simulink model "sixDOF"  (R2023b)
settings: Solver=FixedStepAuto  StartTime=0.0  StopTime=500  FixedStep=time_step  RelTol=1e-3
model workspace: external: MAT-File params.mat (data not in the file)
values from neighbouring files (symbols this model uses):
  currentmass = 0.3    [params.mat]
  drymass = 0.25    [params.mat]    (also in setRocketConstants.m)
  earth_mass = 5.9722e+24    [params.mat]
  earth_radius = 6371852    [params.mat]
  G = 6.6743e-11    [params.mat]
  motor = [0 0.002 0.05 0.1 0.2 0.274 0.292 0.31 0.32 0.33 0.34 0.35 ... (64 elements, 32x2)]    [params.mat]    (also in setRocketConstants.m = table2array(readtable('motor.txt')))
  q0 = [1 0 0 0]    [params.mat]    (also in setRocketConstants.m = [1; 0; 0; 0])
  qBody2IMU = [1 0 0 0]    [params.mat]
  time_step = 0.01    [params.mat]
  wetmass = 0.3    [params.mat]    (also in setRocketConstants.m)
  x0 = [0 0 0 0 0 0 0 0 0]    [params.mat]    (also in setRocketConstants.m = [0; 0; 0; 0; 0; 0; 0; 0; 0])
libraries: aerolibutil x6, shared6dof x1, aerolibnav x1
settings Model: Creator=roger  LastModifiedBy=roger

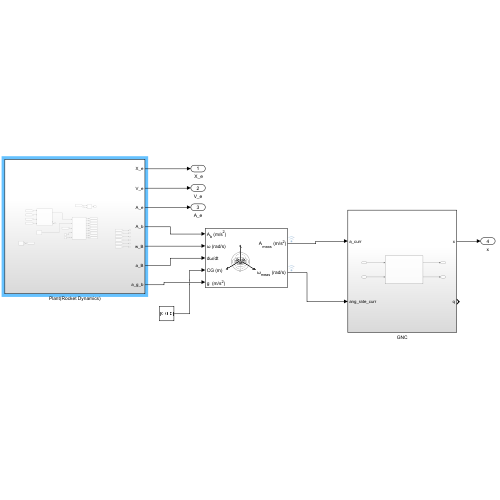
[thumbnail: Simulink's stored preview of the top-level diagram]
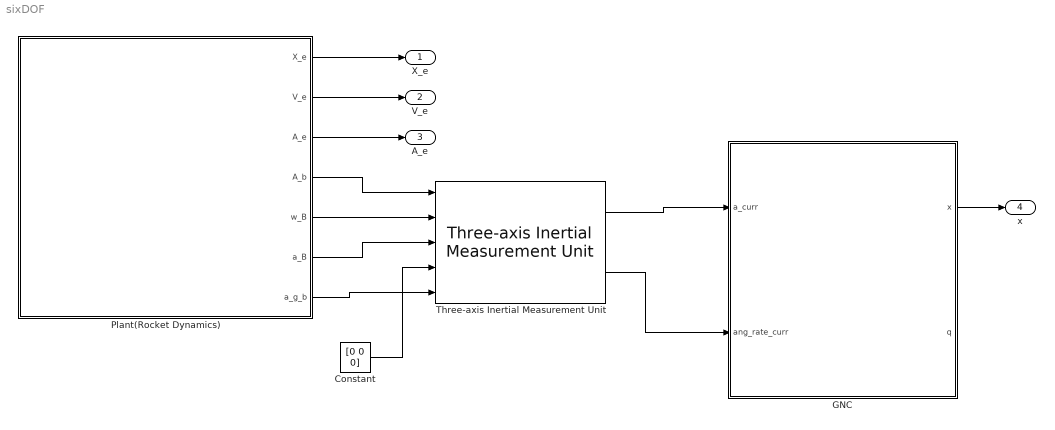
== system sixDOF ==
  Constant : Constant  Value=[0 0 0]
  GNC : Subsystem
  Plant(Rocket Dynamics) : Subsystem
  Three-axis Inertial Measurement Unit : aerolibnav/Three-axis Inertial Measurement Unit  units=Metric (MKS)  imu=[0 0 0]  i_Ts=0.01  dtype_a=on  w_a=190  z_a=0.707  a_sf_cc=[1 0 0; 0 1 0; 0 0 1]  a_bias=[0 0 0]  a_sat="[-inf  -inf  -inf  inf inf inf]"  dtype_g=on  w_g=190  z_g=0.707  g_sf_cc=[1 0 0; 0 1 0; 0 0 1]  g_bias=[0 0 0]  g_sens=[0 0 0]  g_sat="[-inf  -inf  -inf  inf inf inf]"  i_rand=off  i_seeds=[23093 23094 23095 23096 23097 23098]  i_pow=[0.001 0.001 0.001 0.0001 0.0001 0.0001]
  " X_e" : Outport
  V_e : Outport  Port=2
  A_e : Outport  Port=3
  x : Outport  Port=4
  wires:
  Constant/1 -> Three-axis Inertial Measurement Unit/4
  Plant(Rocket Dynamics)/3(A_e) -> A_e/1
  Plant(Rocket Dynamics)/5(w_B) -> Three-axis Inertial Measurement Unit/2
  Plant(Rocket Dynamics)/6(a_B) -> Three-axis Inertial Measurement Unit/3
  Plant(Rocket Dynamics)/4(A_b) -> Three-axis Inertial Measurement Unit/1
  Plant(Rocket Dynamics)/7(a_g_b) -> Three-axis Inertial Measurement Unit/5
  Plant(Rocket Dynamics)/1(X_e) -> " X_e"/1
  Plant(Rocket Dynamics)/2(V_e) -> V_e/1
  Three-axis Inertial Measurement Unit/1 -> GNC/1(a_curr)
  Three-axis Inertial Measurement Unit/2 -> GNC/2(ang_rate_curr)
  GNC/1(x) -> x/1

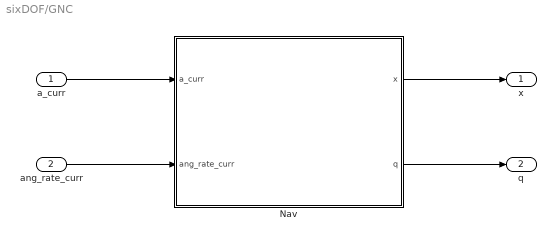
== system sixDOF/GNC ==
  a_curr : Inport
  ang_rate_curr : Inport  Port=2
  Nav : Subsystem
  x : Outport
  q : Outport  Port=2
  wires:
  a_curr/1 -> Nav/1(a_curr)
  ang_rate_curr/1 -> Nav/2(ang_rate_curr)
  Nav/1(x) -> x/1
  Nav/2(q) -> q/1

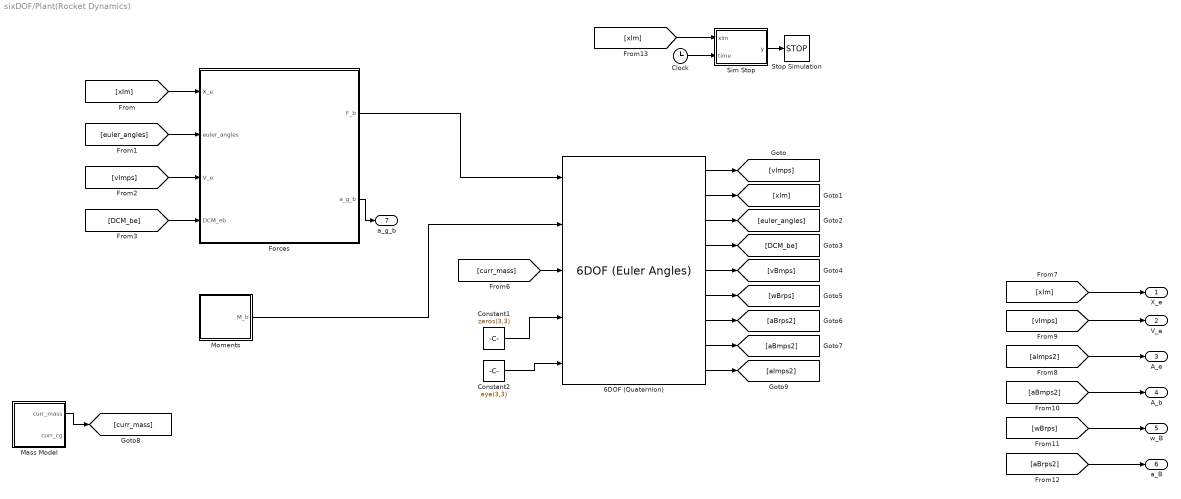
== system sixDOF/Plant(Rocket Dynamics) ==
  "6DOF (Quaternion) " : shared6dof/6DOF (Euler Angles)  units=Metric (MKS)  mtype=Custom Variable  rep=Quaternion  xme_0=[0 0 0]  Vm_0=[0 0 0]  eul_0=[0 0 0]  pm_0=[0 0 0]  mass_0=wetmass  mass_e=drymass  mass_f=wetmass  inertia=eye(3)  inertia_e=eye(3)  inertia_f=2*eye(3)  k_quat=1.0  vre_flag=off  abi_flag=on  aMode=0  xme_statename=''  Vm_statename=''  eul_statename=''  quat_statename=''  pm_statename=''  mass_statename=''
      settings: LibrarySourceBlock=aerolib6dof2/6DOF (Quaternion)
  Clock : Clock
  Constant1 : Constant  Value=zeros(3,3)
  Constant2 : Constant  Value=eye(3,3)
  Forces : Subsystem
  Mass Model : Subsystem
  Moments : Subsystem
  Sim Stop : MATLAB Function  TreatAsAtomicUnit=on
  Stop Simulation : Stop
  X_e : Outport
  V_e : Outport  Port=2
  A_e : Outport  Port=3
  A_b : Outport  Port=4
  w_B : Outport  Port=5
  a_B : Outport  Port=6
  a_g_b : Outport  Port=7
  wires:
  Forces/1(F_b) -> "6DOF (Quaternion) "/1
  Moments/1(M_b) -> "6DOF (Quaternion) "/2
  Constant2/1 -> "6DOF (Quaternion) "/5
  Constant1/1 -> "6DOF (Quaternion) "/4
  [xIm] -> Forces/1(X_e)
  "6DOF (Quaternion) "/1 -> [vImps]
  "6DOF (Quaternion) "/2 -> [xIm]
  "6DOF (Quaternion) "/3 -> [euler_angles]
  "6DOF (Quaternion) "/4 -> [DCM_be]
  "6DOF (Quaternion) "/5 -> [vBmps]
  "6DOF (Quaternion) "/6 -> [wBrps]
  "6DOF (Quaternion) "/7 -> [aBrps2]
  "6DOF (Quaternion) "/8 -> [aBmps2]
  "6DOF (Quaternion) "/9 -> [aImps2]
  [euler_angles] -> Forces/2(euler_angles)
  [vImps] -> Forces/3(V_e)
  [DCM_be] -> Forces/4(DCM_eb)
  Mass Model/1(curr_mass) -> [curr_mass]
  [curr_mass] -> "6DOF (Quaternion) "/3
  [xIm] -> X_e/1
  [aImps2] -> A_e/1
  [vImps] -> V_e/1
  [aBmps2] -> A_b/1
  [wBrps] -> w_B/1
  [aBrps2] -> a_B/1
  Forces/2(a_g_b) -> a_g_b/1
  Clock/1 -> Sim Stop/2(time)
  Sim Stop/1(y) -> Stop Simulation/1
  [xIm] -> Sim Stop/1(xIm)

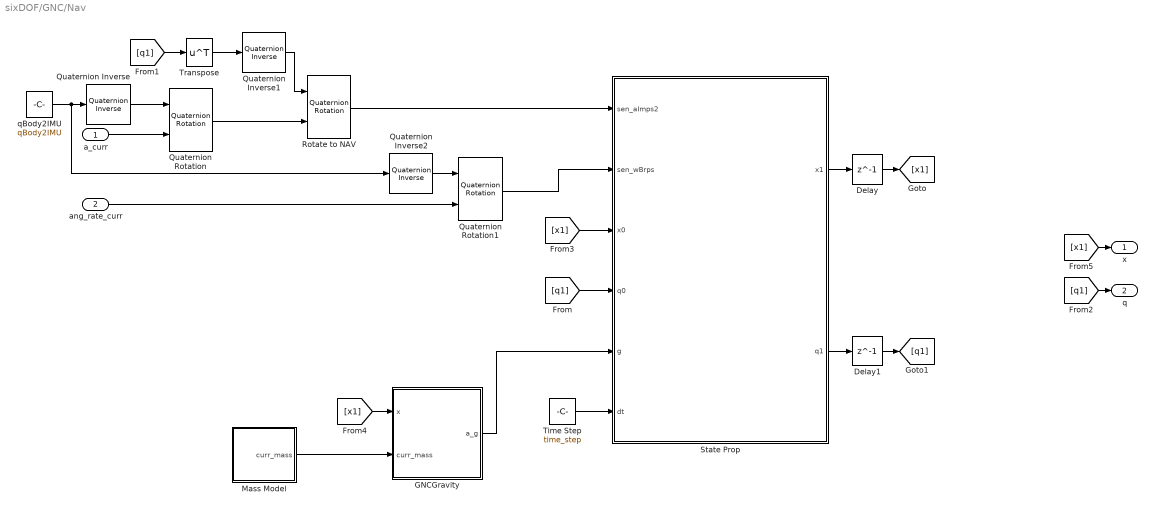
== system sixDOF/GNC/Nav ==
  a_curr : Inport
  ang_rate_curr : Inport  Port=2
  Delay : Delay  DelayLength=1  InitialCondition=x0
  Delay1 : Delay  DelayLength=1  InitialCondition=q0
  GNCGravity : MATLAB Function  TreatAsAtomicUnit=on
  Mass Model : Subsystem
  Quaternion Inverse : aerolibutil/Quaternion Inverse
  Quaternion Inverse1 : aerolibutil/Quaternion Inverse
  Quaternion Inverse2 : aerolibutil/Quaternion Inverse
  Quaternion Rotation : aerolibutil/Quaternion Rotation
  Quaternion Rotation1 : aerolibutil/Quaternion Rotation
  Rotate to NAV : aerolibutil/Quaternion Rotation
  State Prop : MATLAB Function  TreatAsAtomicUnit=on
  Time Step : Constant  Value=time_step
  Transpose : Math  Operator=transpose
  qBody2IMU : Constant  Value=qBody2IMU  VectorParams1D=off
  x : Outport
  q : Outport  Port=2
  wires:
  Time Step/1 -> State Prop/6(dt)
  Transpose/1 -> Quaternion Inverse1/1
  Rotate to NAV/1 -> State Prop/1(sen_aImps2)
  Delay/1 -> [x1]
  State Prop/2(q1) -> Delay1/1
  a_curr/1 -> Quaternion Rotation/2
  Delay1/1 -> [q1]
  GNCGravity/1(a_g) -> State Prop/5(g)
  Quaternion Rotation/1 -> Rotate to NAV/2
  Mass Model/1(curr_mass) -> GNCGravity/2(curr_mass)
  Quaternion Rotation1/1 -> State Prop/2(sen_wBrps)
  Quaternion Inverse2/1 -> Quaternion Rotation1/1
  State Prop/1(x1) -> Delay/1
  Quaternion Inverse1/1 -> Rotate to NAV/1
  qBody2IMU/1 -> Quaternion Inverse2/1, Quaternion Inverse/1
  Quaternion Inverse/1 -> Quaternion Rotation/1
  ang_rate_curr/1 -> Quaternion Rotation1/2
  [q1] -> State Prop/4(q0)
  [q1] -> Transpose/1
  [q1] -> q/1
  [x1] -> State Prop/3(x0)
  [x1] -> GNCGravity/1(x)
  [x1] -> x/1

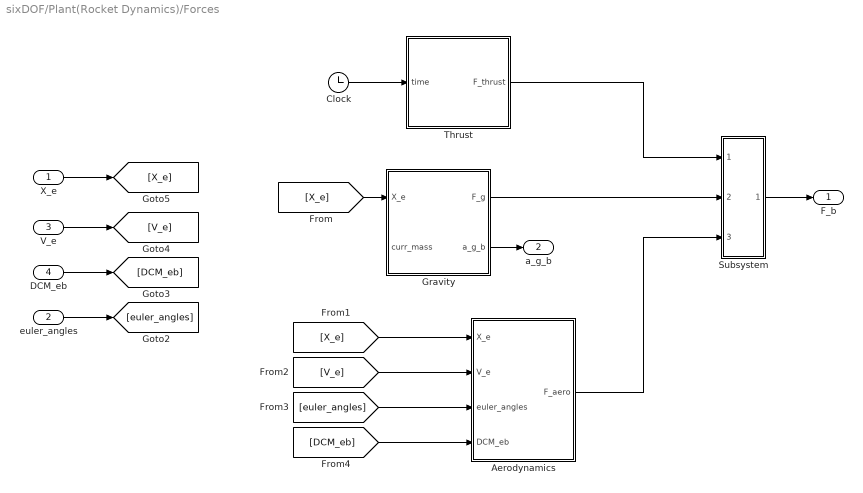
== system sixDOF/Plant(Rocket Dynamics)/Forces ==
  X_e : Inport
  euler_angles : Inport  Port=2
  V_e : Inport  Port=3
  DCM_eb : Inport  Port=4
  Aerodynamics : Subsystem
  Clock : Clock
  Gravity : MATLAB Function  TreatAsAtomicUnit=on
  Subsystem : Subsystem
  Thrust : MATLAB Function  TreatAsAtomicUnit=on
  F_b : Outport
  a_g_b : Outport  Port=2
  wires:
  Clock/1 -> Thrust/1(time)
  Gravity/2(a_g_b) -> a_g_b/1
  euler_angles/1 -> [euler_angles]
  DCM_eb/1 -> [DCM_eb]
  V_e/1 -> [V_e]
  X_e/1 -> [X_e]
  [X_e] -> Gravity/1(X_e)
  [X_e] -> Aerodynamics/1(X_e)
  [V_e] -> Aerodynamics/2(V_e)
  [euler_angles] -> Aerodynamics/3(euler_angles)
  [DCM_eb] -> Aerodynamics/4(DCM_eb)
  Thrust/1(F_thrust) -> Subsystem/1(In1)
  Gravity/1(F_g) -> Subsystem/2(In2)
  Aerodynamics/1(F_aero) -> Subsystem/3(In3)
  Subsystem/1(F_b) -> F_b/1

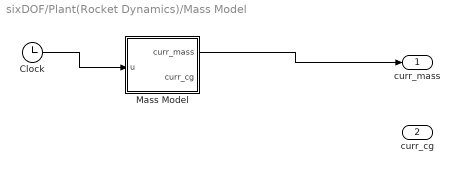
== system sixDOF/Plant(Rocket Dynamics)/Mass Model ==
  Clock : Clock
  Mass Model : MATLAB Function  TreatAsAtomicUnit=on
  curr_mass : Outport
  curr_cg : Outport  Port=2
  wires:
  Mass Model/1(curr_mass) -> curr_mass/1
  Clock/1 -> Mass Model/1(u)

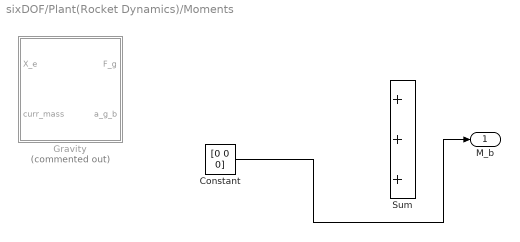
== system sixDOF/Plant(Rocket Dynamics)/Moments ==
  Constant : Constant  Value=[0 0 0]
  Gravity : MATLAB Function  Commented=on  TreatAsAtomicUnit=on
  Sum : Sum  Inputs=+++
  M_b : Outport
  wires:
  Constant/1 -> M_b/1

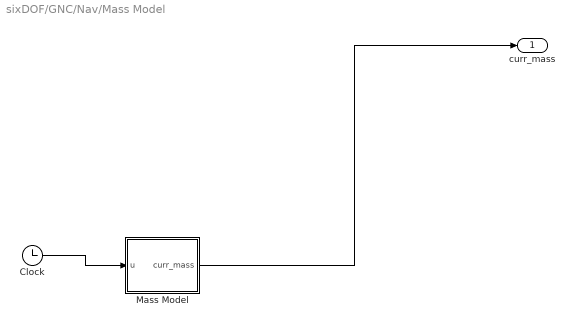
== system sixDOF/GNC/Nav/Mass Model ==
  Clock : Clock
  Mass Model : MATLAB Function  TreatAsAtomicUnit=on
  curr_mass : Outport
  wires:
  Mass Model/1(curr_mass) -> curr_mass/1
  Clock/1 -> Mass Model/1(u)

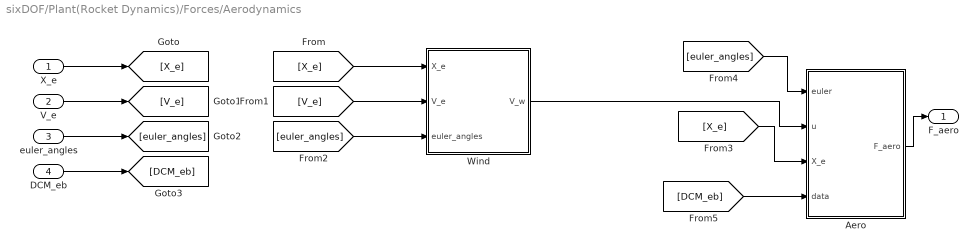
== system sixDOF/Plant(Rocket Dynamics)/Forces/Aerodynamics ==
  X_e : Inport
  V_e : Inport  Port=2
  euler_angles : Inport  Port=3
  DCM_eb : Inport  Port=4
  Aero : MATLAB Function  TreatAsAtomicUnit=on
  Wind : MATLAB Function  TreatAsAtomicUnit=on
  F_aero : Outport
  wires:
  X_e/1 -> [X_e]
  V_e/1 -> [V_e]
  euler_angles/1 -> [euler_angles]
  [X_e] -> Wind/1(X_e)
  [V_e] -> Wind/2(V_e)
  [euler_angles] -> Wind/3(euler_angles)
  Wind/1(V_w) -> Aero/2(u)
  [X_e] -> Aero/3(X_e)
  Aero/1(F_aero) -> F_aero/1
  [euler_angles] -> Aero/1(euler)
  DCM_eb/1 -> [DCM_eb]
  [DCM_eb] -> Aero/4(data)

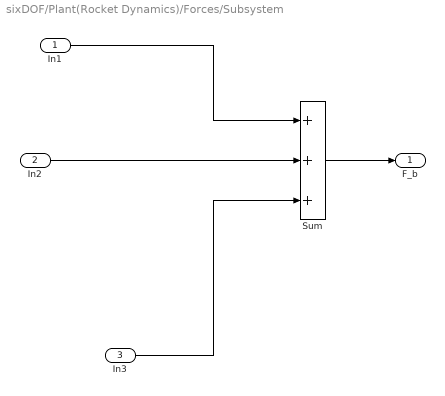
== system sixDOF/Plant(Rocket Dynamics)/Forces/Subsystem ==
  In1 : Inport
  In2 : Inport  Port=2
  In3 : Inport  Port=3
  Sum : Sum  Inputs=+++
  F_b : Outport
  wires:
  Sum/1 -> F_b/1
  In3/1 -> Sum/3
  In1/1 -> Sum/1
  In2/1 -> Sum/2

== matlab function sixDOF/Plant(Rocket Dynamics)/Mass Model/Mass Model ==
  data: u input; curr_mass output; wetmass parameter; drymass parameter; curr_cg output
function [curr_mass, curr_cg]= fcn(u, wetmass, drymass)

curr_mass = wetmass;
curr_cg = 5;

== matlab function sixDOF/GNC/Nav/GNCGravity ==
  data: x input; curr_mass input; G parameter; earth_mass parameter; earth_radius parameter; a_g output
function a_g = fcn(x, curr_mass, G, earth_mass, earth_radius)

g = G * earth_mass / ((earth_radius + x(3)) ^ 2);

a_g = [0, 0, g];

== matlab function sixDOF/GNC/Nav/Mass Model/Mass Model ==
  data: u input; curr_mass output; wetmass parameter; drymass parameter
function curr_mass = fcn(u, wetmass, drymass)

curr_mass = wetmass;

== matlab function sixDOF/Plant(Rocket Dynamics)/Forces/Aerodynamics/Aero ==
  data: euler input; u input; F_aero output; X_e input; data input
function F_aero = fcn(euler, u, X_e, data)

F_aero = u;

== matlab function sixDOF/Plant(Rocket Dynamics)/Forces/Aerodynamics/Wind ==
  data: X_e input; V_e input; V_w output; currentmass parameter; euler_angles input
function V_w = fcn(X_e, V_e, currentmass, euler_angles)



%{
steps:
find wind velocities
add to V_e to get V_air


aero considerations:
wind

forces summed
Cn(up), Ca(long), Cy(side)
Cl, Cd

A cos a
%}



V_w = [0, 0, 0];

== matlab function sixDOF/Plant(Rocket Dynamics)/Forces/Thrust ==
  data: time input; F_thrust output; motor parameter; currentmass parameter; drymass parameter; wetmass parameter
function F_thrust = fcn(time, motor, currentmass, drymass, wetmass)

if time < 2.44 
    currentmass = wetmass - ((wetmass - drymass)/(2.44)) * (time);
    N = interp1(motor(:, 1), motor(:, 2), time);
else
    N = 0;
end 
F_thrust = [0, 0, N];

== matlab function sixDOF/Plant(Rocket Dynamics)/Forces/Gravity ==
  data: X_e input; F_g output; curr_mass input; G parameter; earth_mass parameter; earth_radius parameter; a_g_b output
function [F_g, a_g_b]= fcn(X_e, curr_mass, G, earth_mass, earth_radius)

g = G * earth_mass / ((earth_radius + X_e(3)) ^ 2);

F_g = [0, 0,  - g * curr_mass]; 

a_g_b = [0 , 0, g];

== matlab function sixDOF/GNC/Nav/State Prop ==
  data: x1 output; sen_aImps2 input; sen_wBrps input; x0 input; q0 input; g input; q1 output; dt input
function [x1, q1] = fcn(sen_aImps2, sen_wBrps, x0, q0, g, dt)
 %{
    Purpose:
        Propagates state vector given sensor outputs 
    Parameters:
        aSensor (1 x 3 Matrix): Acceleration IMU output
        wSensor (1 x 3 Matrix): Angular velocity IMU output
        x0 (9 x 1 Matrix): Translational position/velocity/acceleration state vector
        q0 (4 x 1 Matrix): Orientation quaternion state vector
        dt (float): Time step in s
        g: accel due to gravity(temp)
    
    Returns:
        x1: 9 x 1 State vector
        q1: aSensor: 4 x 1 quaternion matrix
 %}
    %%need to write the custom quaternion functions:quatrotate, quatinv
    %correct for gravity
   
    sen_aImps2 = sen_aImps2 + g.';
    x1 = propPos(x0, sen_aImps2, dt);
    q1 = propAtt(q0, sen_wBrps, dt);
  
end

function [x1] = propPos(x0, a, dt)
    
    F = [
        1, 0, 0, dt, 0, 0, (dt^2)/2, 0, 0;
        0, 1, 0, 0, dt, 0, 0, (dt^2)/2, 0;
        0, 0, 1, 0, 0, dt, 0, 0, (dt^2)/2;

        0, 0, 0, 1, 0, 0, dt, 0, 0;
        0, 0, 0, 0, 1, 0, 0, dt, 0;
        0, 0, 0, 0, 0, 1, 0, 0, dt;

        0, 0, 0, 0, 0, 0, 1, 0, 0;
        0, 0, 0, 0, 0, 0, 0, 1, 0;
        0, 0, 0, 0, 0, 0, 0, 0, 1;
        ];
    x1 = F * x0;
    x1(7:end, 1) = a.';
end

function [q1] = propAtt(q0, w, dt)
    q1 = ((eye(4) + (1/2) * omega(w) * dt) * q0);
    q1 = q1/norm(q1);
end

function [o] = omega(w)
    o = [0 -w(1) -w(2) -w(3);
        w(1) 0 w(3) -w(2);
        w(2) -w(3) 0 w(1);
        w(3) w(2) -w(1) 0];
end

== matlab function sixDOF/Plant(Rocket Dynamics)/Sim Stop ==
  data: xIm input; y output; time input
function y = fcn(xIm, time)

if time > 10 & xIm(3) < 0
    y = 1;
else 
    y = 0;
end

== matlab function sixDOF/Plant(Rocket Dynamics)/Moments/Gravity ==
  data: X_e input; F_g output; curr_mass input; G parameter; earth_mass parameter; earth_radius parameter; a_g_b output
function [F_g, a_g_b]= fcn(X_e, curr_mass, G, earth_mass, earth_radius)

g = G * earth_mass / ((earth_radius + X_e(3)) ^ 2);

F_g = [0, 0,  - g * curr_mass]; 

a_g_b = [0 , 0, g];
